simulink model "Problem2"  (Simulink 8.6)
settings: Solver=VariableStepAuto  StartTime=0.0  StopTime=24  RelTol=1e-3
settings Model: Creator=Nikki  LastModifiedBy=Nikki
settings DataIOCC: SaveFormat=Dataset  SignalLoggingSaveFormat=Dataset
settings OptimizationCC: ExpressionDepthLimit=128
settings DebuggingCC: UnderspecifiedInitializationDetection=Simplified  MergeDetectMultiDrivingBlocksExec=error  SolverPrmCheckMsg=none  FcnCallInpInsideContextMsg=EnableAllAsError  StateNameClashWarn=none
settings HardwareCC: ProdBitPerPointer=64  ProdLargestAtomicFloat=Float  ProdIntDivRoundTo=Zero  ProdEndianess=LittleEndian  ProdWordSize=64  ProdHWDeviceType=Intel->x86-64 (Windows64)
settings GRTTargetCC: GeneratePreprocessorConditionals=Use local settings  CombineOutputUpdateFcns=on  GRTInterface=off
settings ConfigComp: CovModelRefEnable=off

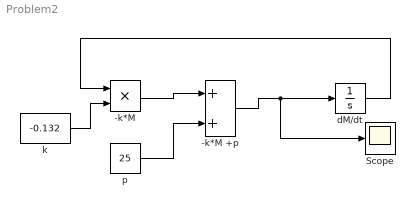
== system Problem2 ==
  -k*M : Product
  -k*M +p : Sum
  Scope : Scope
  dM/dt : Integrator
  k : Constant  Value=-0.132  VectorParams1D=off
  p : Constant  Value=25
  wires:
  k/1 -> -k*M/2
  dM/dt/1 -> -k*M/1
  -k*M/1 -> -k*M +p/1
  p/1 -> -k*M +p/2
  -k*M +p/1 -> Scope/1, dM/dt/1
